simulink model "Xplained_SAMx7_EEPROM_EFC_R2020b"  (R2020b)
settings: Solver=FixedStepDiscrete  StartTime=0.0  StopTime=10.0  FixedStep=0.001  RelTol=1e-3  EnableMultiTasking=on
model workspace (MAT data in the model file):
  EEPROM_0x45_0000 : Simulink.Signal (value not decoded)
symbols that are objects in the model workspace (value not decoded): EEPROM_0x45_0000
undefined symbols (not defined in the file): DiscIntNeverNeededParam, LQFP144, SAME70Q21B, Timer
libraries: MCHP_Blockset x8, simulink x6, simulink_extras x1
(part 2 of 2)

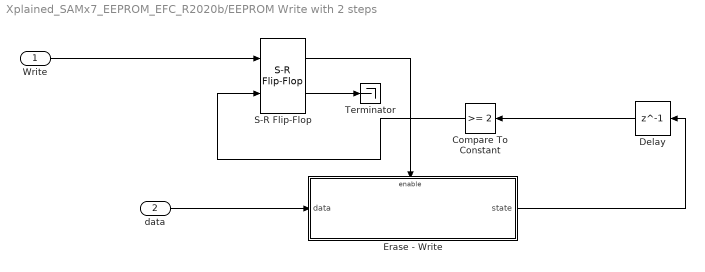
== system Xplained_SAMx7_EEPROM_EFC_R2020b/EEPROM Write with 2 steps ==
  Write : Inport
  data : Inport  Port=2
  Compare To Constant : simulink/Logic and Bit Operations/Compare To Constant  relop=>=  const=2  OutDataTypeStr=boolean
  Delay : Delay  DelayLength=1  InitialCondition=0
  Erase - Write : Subsystem
  S-R Flip-Flop : simulink_extras/Flip Flops/S-R Flip-Flop  initial_condition=0
  Terminator : Terminator
  wires:
  Erase - Write/1(state) -> Delay/1
  Write/1 -> S-R Flip-Flop/1
  Compare To Constant/1 -> S-R Flip-Flop/2
  data/1 -> Erase - Write/1(data)
  S-R Flip-Flop/2 -> Terminator/1
  Delay/1 -> Compare To Constant/1
  S-R Flip-Flop/1 -> Erase - Write/Enable

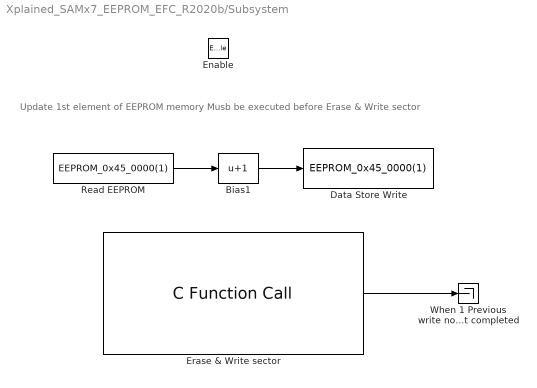
== system Xplained_SAMx7_EEPROM_EFC_R2020b/Subsystem ==
  note: Update 1st element of EEPROM memory
      | Musb be executed before Erase & Write sector
  Enable : EnablePort
  Bias1 : Bias  Bias=1
  Data Store Write : DataStoreWrite  Priority=-2000  DataStoreName=EEPROM_0x45_0000  DataStoreElements=EEPROM_0x45_0000(1)
  Erase & Write sector : MCHP_Blockset/User Functions/C Function Call  Priority=100  ParseFilesChkbx=on  ListFunctions1=Custom Function  Function1=int EFC_PageEraseWrite(uint32_t address)  AddHeaderDeclaration=on  Function1Type=when block is updated (default)  Fct1BlockIn=address=0x450000  FctReturnBlockOut=on  DataCollected="s.chksm={ '706715-sept.-2021 11:02:20'};s.File1=reshape({ '  int  EFC_PageEraseWrite(uint32_t address)','  void  EFC_Handler(void)'},1,2);"  ORDERING=None  SampleTime=-1  S_INPUT=0  S_INPUT_Size=0  S_OUTPUT=0  S_OUTPUT_Size=0  S_ListCustomDatatype=0  MCHP_CRC=1014111  MCHP_MASTERLINK=Xplained_SAMx7_EEPROM_EFC_R2020b/Microchip Master  PinDigitalInput=[]  PinDigitalOutput=[]  PinAnalogInput=[]
      settings: SourceProductName=MPLAB Device Blocks for Simulink
  Read EEPROM : DataStoreRead  DataStoreName=EEPROM_0x45_0000  DataStoreElements=EEPROM_0x45_0000(1)
  "When 1 Previous write not completed " : Terminator
  wires:
  Erase & Write sector/1 -> "When 1 Previous write not completed "/1
  Read EEPROM/1 -> Bias1/1
  Bias1/1 -> Data Store Write/1

== system Xplained_SAMx7_EEPROM_EFC_R2020b/WWW Xplained User Guide ==

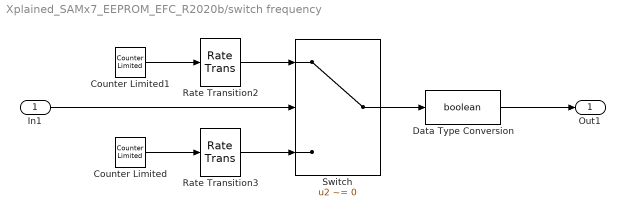
== system Xplained_SAMx7_EEPROM_EFC_R2020b/switch frequency ==
  In1 : Inport
  Counter Limited : simulink/Sources/Counter Limited  uplimit=1  tsamp=.2
  Counter Limited1 : simulink/Sources/Counter Limited  uplimit=1  tsamp=.1
  Data Type Conversion : DataTypeConversion  OutDataTypeStr=boolean
  Rate Transition2 : RateTransition
  Rate Transition3 : RateTransition
  Switch : Switch  Criteria=u2 ~= 0
  Out1 : Outport
  wires:
  Rate Transition2/1 -> Switch/1
  Switch/1 -> Data Type Conversion/1
  Counter Limited1/1 -> Rate Transition2/1
  Rate Transition3/1 -> Switch/3
  Counter Limited/1 -> Rate Transition3/1
  Data Type Conversion/1 -> Out1/1
  In1/1 -> Switch/2

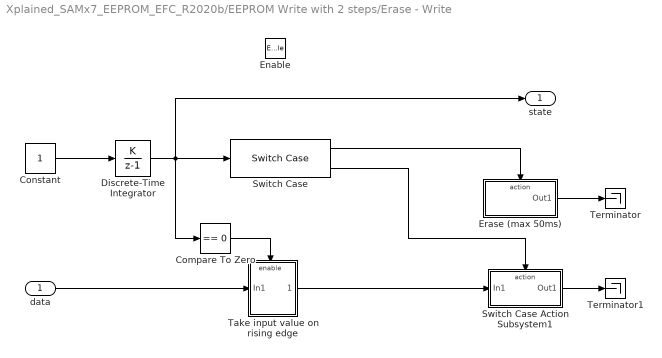
== system Xplained_SAMx7_EEPROM_EFC_R2020b/EEPROM Write with 2 steps/Erase - Write ==
  data : Inport
  Enable : EnablePort  StatesWhenEnabling=reset
  Compare To Zero : simulink/Logic and Bit Operations/Compare To Zero  relop===  OutDataTypeStr=boolean
  Constant : Constant  SampleTime=0.05
  Discrete-Time Integrator : DiscreteIntegrator  IntegratorMethod=Accumulation: Forward Euler  gainval=1  SampleTime=-1  OutDataTypeStr=uint16  SaturateOnIntegerOverflow=on  ICPrevOutput=DiscIntNeverNeededParam  ICPrevScaledInput=DiscIntNeverNeededParam
  Erase (max 50ms) : Subsystem  TreatAsAtomicUnit=on
  Switch Case : SwitchCase  CaseConditions={0,1}  ShowDefaultCase=off
  Switch Case Action Subsystem1 : Subsystem  TreatAsAtomicUnit=on
  "Take input value on rising edge " : Subsystem  TreatAsAtomicUnit=on
  Terminator : Terminator
  Terminator1 : Terminator
  state : Outport  OutputWhenDisabled=reset  InitialOutput=0
  wires:
  data/1 -> "Take input value on rising edge "/1(In1)
  Constant/1 -> Discrete-Time Integrator/1
  Switch Case/1 -> Erase (max 50ms)/Action
  Discrete-Time Integrator/1 -> state/1, Compare To Zero/1, Switch Case/1
  Switch Case/2 -> Switch Case Action Subsystem1/Action
  Erase (max 50ms)/1(Out1) -> Terminator/1
  Switch Case Action Subsystem1/1(Out1) -> Terminator1/1
  "Take input value on rising edge "/1(Out1) -> Switch Case Action Subsystem1/1(In1)
  Compare To Zero/1 -> "Take input value on rising edge "/Enable

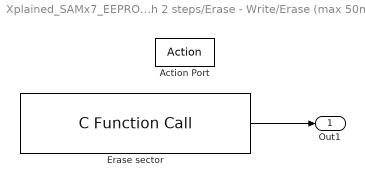
== system Xplained_SAMx7_EEPROM_EFC_R2020b/EEPROM Write with 2 steps/Erase - Write/Erase (max 50ms) ==
  Action Port : ActionPort
  Erase sector : MCHP_Blockset/User Functions/C Function Call  ParseFilesChkbx=on  ListFunctions1=Custom Function  Function1=bool EFC_SectorErase(uint32_t address)  AddHeaderDeclaration=off  Function1Type=when block is updated (default)  Fct1BlockIn=address=0x450000  FctReturnBlockOut=on  DataCollected="s.chksm=reshape({ '469430-juil.-2021 10:06:12','331519-févr.-2021 14:24:16'},1,2);s.File1=reshape({ '  void  EFC_Initialize(void)','  bool  EFC_Read(uint32_t *data, uint32_t length, uint32_t address)','  bool  EFC_SectorErase(uint32_t address)','  bool  EFC_PageWrite(uint32_t *data, uint32_t address)','  bool  EFC_QuadWordWrite(uint32_t *data, uint32_t address)','  void  EFC_RegionLock(uint32_t address)','  void  EFC_RegionUnlock(uint32_t address)','  bool  EFC_IsBusy(void)'},1,8);s.File2={};"  ORDERING=None  SampleTime=-1  S_INPUT=0  S_INPUT_Size=0  S_OUTPUT=0  S_OUTPUT_Size=0  S_ListCustomDatatype=0  MCHP_CRC=1343969  MCHP_MASTERLINK=Xplained_SAMx7_EEPROM_EFC_R2020b/Microchip Master  PinDigitalInput=[]  PinDigitalOutput=[]  PinAnalogInput=[]
      settings: SourceProductName=MPLAB Device Blocks for Simulink
  Out1 : Outport
  wires:
  Erase sector/1 -> Out1/1

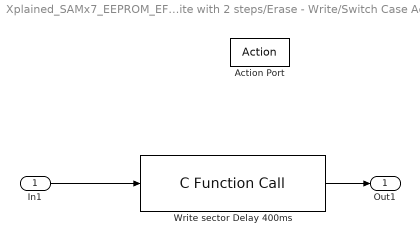
== system Xplained_SAMx7_EEPROM_EFC_R2020b/EEPROM Write with 2 steps/Erase - Write/Switch Case Action Subsystem1 ==
  In1 : Inport
  Action Port : ActionPort
  "Write sector Delay 400ms " : MCHP_Blockset/User Functions/C Function Call  ParseFilesChkbx=on  ListFunctions1=Custom Function  Function1=bool EFC_PageWrite(uint32_t *data, uint32_t address)  AddHeaderDeclaration=off  Function1Type=when block is updated (default)  Fct1BlockIn="data[512]  , address=0x450000"  FctReturnBlockOut=on  DataCollected="s.chksm=reshape({ '469630-juil.-2021 09:29:03','331519-févr.-2021 14:24:16'},1,2);s.File1=reshape({ '  void  EFC_Initialize(void)','  bool  EFC_Read(uint32_t *data, uint32_t length, uint32_t address)','  bool  EFC_SectorErase(uint32_t address)','  bool  EFC_PageWrite(uint32_t *data, uint32_t address)','  bool  EFC_QuadWordWrite(uint32_t *data, uint32_t address)','  void  EFC_RegionLock(uint32_t address)','  void  EFC_RegionUnlock(uint32_t address)','  bool  EFC_IsBusy(void)'},1,8);s.File2={};"  ORDERING=None  SampleTime=-1  S_INPUT=0  S_INPUT_Size=0  S_OUTPUT=0  S_OUTPUT_Size=0  S_ListCustomDatatype=0  MCHP_CRC=1368873  MCHP_MASTERLINK=Xplained_SAMx7_EEPROM_EFC_R2020b/Microchip Master  PinDigitalInput=[]  PinDigitalOutput=[]  PinAnalogInput=[]
      settings: SourceProductName=MPLAB Device Blocks for Simulink
  Out1 : Outport
  wires:
  In1/1 -> "Write sector Delay 400ms "/1
  "Write sector Delay 400ms "/1 -> Out1/1

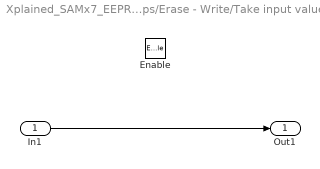
== system Xplained_SAMx7_EEPROM_EFC_R2020b/EEPROM Write with 2 steps/Erase - Write/Take input value on rising edge  ==
  In1 : Inport
  Enable : EnablePort
  Out1 : Outport
  wires:
  In1/1 -> Out1/1
